simulink library "Batt_lib"  (Simulink 7.8)
settings: Solver=ode45  StartTime=0.0  StopTime=10.0  RelTol=1e-3
values from neighbouring files (symbols this model uses):
  batt_esr = (max_power*0.01)/(max_power/Vdc_nom)^2    [BES_init.m]
  C = IacRMS*18e-6    [BES_init.m]
  f = 60    [global_parameters.m]
  I_ki = 0.03    [BES_init.m]
  I_kp = 0.05    [BES_init.m]
  Iac_max = IGBT_currents(possible_currents(1))    [BES_init.m]
  Id_at_max = 3*max_pow*(2/3)/Vd_at_max    [BES_init.m]
  Iq_at_max = 3*max_pow*(2/3)/Vq_at_max    [BES_init.m]
  L = Vdc_nom/(IacRMS*0.2/(2/fs))    [BES_init.m]
  PLL_Ki = 0.001*30    (= 0.03)    [BES_init.m]
  PLL_Kp = .001*30    (= 0.03)    [BES_init.m]
  PLL_time_step = Ts    (= 8e-05)    [global_parameters.m]
  Roff = 1e7    (= 10000000)    [BES_init.m]
  Td_es_min = Ts    (= 8e-05)    [global_parameters.m]
  Tds = Ts    (= 8e-05)    [global_parameters.m]
  Ts = 80e-6    (= 8e-05)    [global_parameters.m]    (also in scopeBuffer.m)
  Vdc_max = IGBT_voltages(possible_voltages(1))    [BES_init.m]
undefined symbols (not defined in the file or in its folder): D, DiscIntNeverNeededParam
libraries: powerlib x17, simulink x14, simulink_extras x8, cstextras x3, rtio_generic_modbus x1, powerlib_extras x1
settings Model: Creator=re25624  LastModifiedBy=RE25624

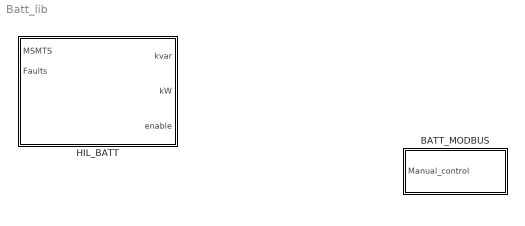
== system Batt_lib ==
  BATT_MODBUS : Subsystem
  HIL_BATT : Subsystem

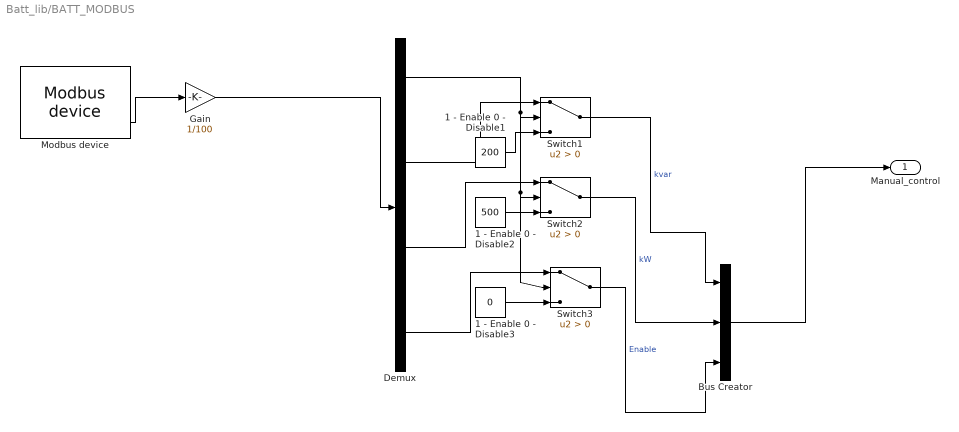
== system Batt_lib/BATT_MODBUS ==
  1 - Enable 0 - Disable1 : Constant  Value=200
  1 - Enable 0 - Disable2 : Constant  Value=500
  1 - Enable 0 - Disable3 : Constant  Value=0
  Bus Creator : BusCreator  Inputs=3
  Demux : Demux
  Gain : Gain  Gain=1/100
  Modbus device : rtio_generic_modbus/Modbus device  conf_name=batt_slave_cfg.opal  conf_name_mask=batt_slave_cfg.xls  sample_time=Ts
  Switch1 : Switch  Criteria=u2 > Threshold
  Switch2 : Switch  Criteria=u2 > Threshold
  Switch3 : Switch  Criteria=u2 > Threshold
  Manual_control : Outport
  wires:
  Bus Creator/1 -> Manual_control/1
  Switch3/1 -> Bus Creator/3  "Enable"
  Switch2/1 -> Bus Creator/2  "kW"
  Switch1/1 -> Bus Creator/1  "kvar"
  Demux/1 -> Switch3/2, Switch2/2, Switch1/2
  Demux/4 -> Switch3/1
  Demux/3 -> Switch2/1
  Demux/2 -> Switch1/1
  1 - Enable 0 - Disable3/1 -> Switch3/3
  1 - Enable 0 - Disable2/1 -> Switch2/3
  1 - Enable 0 - Disable1/1 -> Switch1/3
  Gain/1 -> Demux/1
  Modbus device/2 -> Gain/1

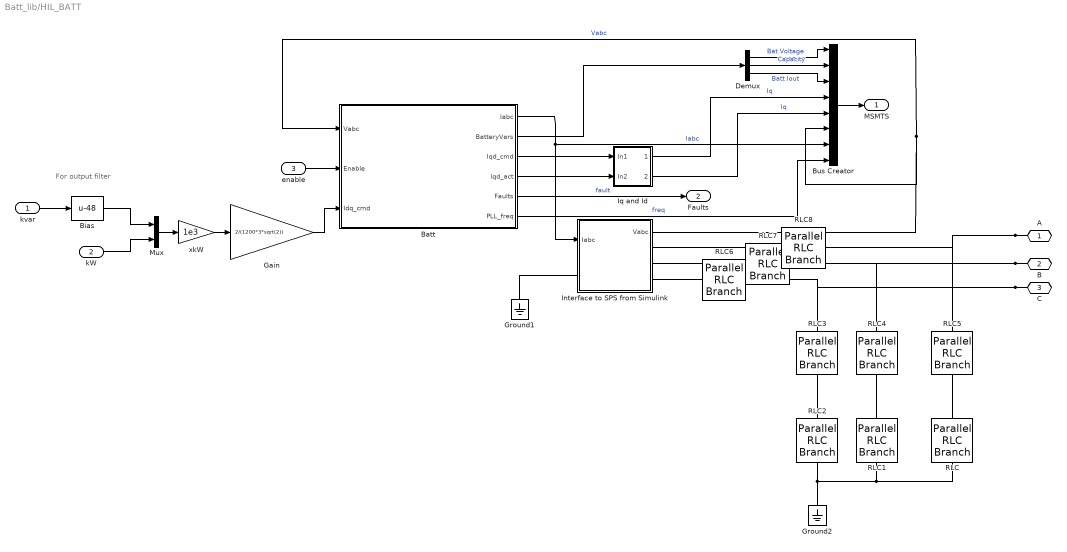
== system Batt_lib/HIL_BATT ==
  note: For output filter
  kvar : Inport
  kW : Inport  Port=2
  enable : Inport  Port=3
  Batt : Subsystem  mask(Battery Energy Storage System with AC inverter and Droop Control){max_power=4e6, batt_kWh=500, VacRMS=1200, Vdc_nom=4000}
      mask prompts: max_power "Peak Power (W)"; batt_kWh "Capacity (kWh)"; VacRMS "Grid Tie Line to Neutral Voltage (RMS)"; Vdc_nom "Nominal DC Battery Voltage"
      mask help: The block implements a battery energy storage system suitable for connecting to the grid. It responds to grid voltage changes by injecting current into the grid. The model is a non-switching average model.
      mask init:
      | global_parameters
      | BES_init
      mask Help:
      | This block will likely need a filter and transformer on it's output in order to connect to a high power line.
      | 
      | A unit delay block  on the Iabc output can help remove algebraic loops with minimal impact on simulation results.
      | 
      | 
      | Block Parameters:
      | Peak Power- Maximum power the unit can transfer.
      | Capacity- Amount of energy in the battery.
      | Grid Tie Line to Neutral Voltage- RMS voltage for the grid tie interface.
      | Nominal DC Battery Voltage- Open circuit full charge voltage.
      | Real Power Droop Gain- Ratio of Watts to Hz for injecting power to the grid in response to frequency changes.
      | Reactive Power Droop Gain- Ratio of kVars to RMS volts for injecting reactive power to the grid.
      | Droop Filter Cut Off- Fastest frequency that will be responded to for injecting power to the grid.
      | 
      | 
      | Block Connections:
      | Vabc- Grid voltage for each of the three phases.
      | Enable- Set to zero for no power.  Set to 1 to enable energy tranfer.
      | Iabc- Grid current for each of the three phases.  Connect to your grid.  Positive is into the grid.
      | Battery_vars- A vector of battery voltage, capacity, and current out of the battery.
      | Iqd_cmd- Commanded q and d axis currents.
      | Iqd_act- Actual q and d axis currents.
      mask Display:
      | image(imread('grid_storage_battery.jpg'))
      | color('white')
      | fprintf('%d kW Peak', max_power/1e3)
      | color('black')
      | port_label('input',1,'Vabc')
      | port_label('input',2,'Enable')
      | port_label('input',3,'Idq_cmd')
      | port_label('output',1,'Iabc')
      | port_label('output',2,'Battery_vars')
      | port_label('output',3,'Iqd_cmd')
      | port_label('output',4,'Iqd_act')
      | port_label('output',5,'Faults')
      | port_label('output',6,'Freq')
  Bias : Bias  Bias=-48
  Bus Creator : BusCreator  Inputs=8
  Demux : Demux  Outputs=3
  Gain : Gain  Gain=2/(1200*3*sqrt(2))
  Ground1 : powerlib/Elements/Ground  LConnTagsString=a
  Ground2 : powerlib/Elements/Ground  LConnTagsString=a
  Interface to SPS from Simulink : Subsystem
  Iq and Id : Subsystem
  Mux : Mux  Inputs=2
  "RLC " : powerlib/Elements/Parallel RLC Branch  LConnTagsString=a  RConnTagsString=__new0  BranchType=RLC  Resistance=500  Inductance=inf  SetiL0=off  InitialCurrent=0  Capacitance=10e-6  Setx0=off  InitialVoltage=0  Measurements=None
  RLC1 : powerlib/Elements/Parallel RLC Branch  LConnTagsString=a  RConnTagsString=__new0  BranchType=RLC  Resistance=500  Inductance=inf  SetiL0=off  InitialCurrent=0  Capacitance=10e-6  Setx0=off  InitialVoltage=0  Measurements=None
  RLC2 : powerlib/Elements/Parallel RLC Branch  LConnTagsString=a  RConnTagsString=__new0  BranchType=RLC  Resistance=500  Inductance=inf  SetiL0=off  InitialCurrent=0  Capacitance=10e-6  Setx0=off  InitialVoltage=0  Measurements=None
  RLC3 : powerlib/Elements/Parallel RLC Branch  LConnTagsString=a  RConnTagsString=__new0  BranchType=R  Resistance=10e-3  Inductance=inf  SetiL0=off  InitialCurrent=0  Capacitance=0  Setx0=off  InitialVoltage=0  Measurements=None
  RLC4 : powerlib/Elements/Parallel RLC Branch  LConnTagsString=a  RConnTagsString=__new0  BranchType=R  Resistance=10e-3  Inductance=inf  SetiL0=off  InitialCurrent=0  Capacitance=0  Setx0=off  InitialVoltage=0  Measurements=None
  RLC5 : powerlib/Elements/Parallel RLC Branch  LConnTagsString=a  RConnTagsString=__new0  BranchType=R  Resistance=10e-3  Inductance=inf  SetiL0=off  InitialCurrent=0  Capacitance=0  Setx0=off  InitialVoltage=0  Measurements=None
  RLC6 : powerlib/Elements/Parallel RLC Branch  LConnTagsString=a  RConnTagsString=__new0  BranchType=R  Resistance=20e-3  Inductance=inf  SetiL0=off  InitialCurrent=0  Capacitance=0  Setx0=off  InitialVoltage=0  Measurements=None
  RLC7 : powerlib/Elements/Parallel RLC Branch  LConnTagsString=a  RConnTagsString=__new0  BranchType=R  Resistance=20e-3  Inductance=inf  SetiL0=off  InitialCurrent=0  Capacitance=0  Setx0=off  InitialVoltage=0  Measurements=None
  RLC8 : powerlib/Elements/Parallel RLC Branch  LConnTagsString=a  RConnTagsString=__new0  BranchType=R  Resistance=20e-3  Inductance=inf  SetiL0=off  InitialCurrent=0  Capacitance=0  Setx0=off  InitialVoltage=0  Measurements=None
  xkW : Gain  Gain=1e3
  A : PMIOPort  Port=1  Side=Right
  B : PMIOPort  Port=2  Side=Right
  C : PMIOPort  Port=3  Side=Right
  MSMTS : Outport
  Faults : Outport  Port=2
  wires:
  Batt/5(Faults) -> Faults/1  "fault"
  Interface to SPS from Simulink/1(Vabc) -> Batt/1(Vabc), Bus Creator/6  "Vabc"
  Batt/2(BatteryVars) -> Demux/1
  Demux/2 -> Bus Creator/2  "Capacity"
  Demux/3 -> Bus Creator/3  "Batt Iout"
  Demux/1 -> Bus Creator/1  "Bat Voltage"
  Batt/3(Iqd_cmd) -> Iq and Id/1(In1)
  Batt/4(Iqd_act) -> Iq and Id/2(In2)
  Iq and Id/1(Out1) -> Bus Creator/4  "Iq"
  enable/1 -> Batt/2(Enable)
  Batt/1(Iabc) -> Bus Creator/7, Interface to SPS from Simulink/1(Iabc)  "Iabc"
  Gain/1 -> Batt/3(Idq_cmd)
  xkW/1 -> Gain/1
  Mux/1 -> xkW/1
  Iq and Id/2(Out2) -> Bus Creator/5  "Iq"
  Bus Creator/1 -> MSMTS/1
  kvar/1 -> Bias/1
  kW/1 -> Mux/2
  Batt/6(PLL_freq) -> Bus Creator/8  "freq"
  Bias/1 -> Mux/1
  connections:
  Interface to SPS from Simulink/LConn1 -- Ground1/LConn1
  Ground2/LConn1 -- RLC2/RConn1 -- "RLC "/RConn1 -- RLC1/RConn1
  A/RConn1 -- RLC8/LConn1 -- RLC5/LConn1
  B/RConn1 -- RLC7/LConn1 -- RLC4/LConn1
  C/RConn1 -- RLC6/LConn1 -- RLC3/LConn1
  RLC3/RConn1 -- RLC2/LConn1
  RLC4/RConn1 -- RLC1/LConn1
  RLC5/RConn1 -- "RLC "/LConn1
  RLC6/RConn1 -- Interface to SPS from Simulink/RConn3
  Interface to SPS from Simulink/RConn2 -- RLC7/RConn1
  Interface to SPS from Simulink/RConn1 -- RLC8/RConn1

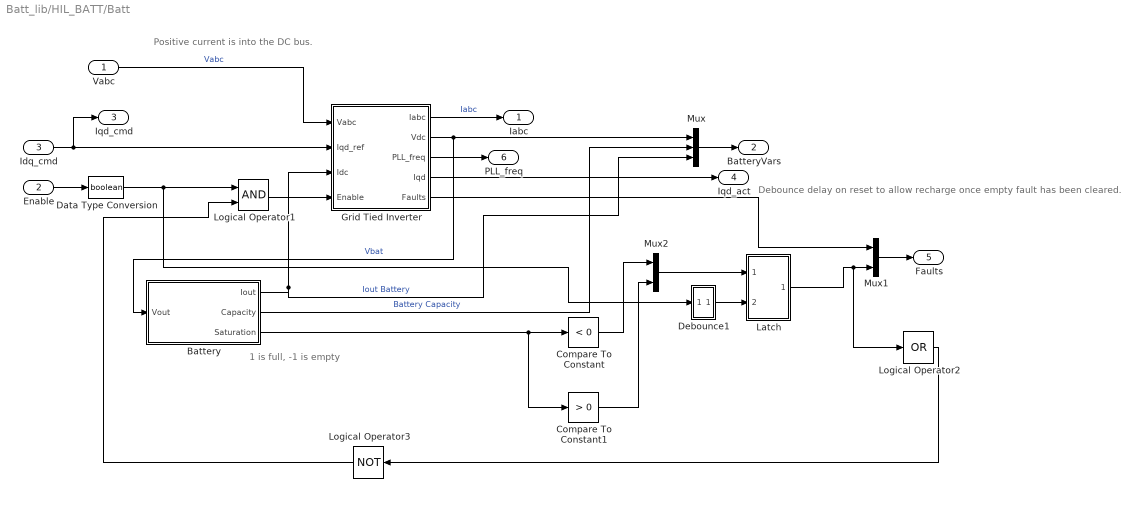
== system Batt_lib/HIL_BATT/Batt ==
  note: Debounce delay on reset to allow recharge once empty fault has been cleared.
  note: 1 is full, -1 is empty
  note: Positive current is into the DC bus.
  Vabc : Inport
  Enable : Inport  Port=2  OutDataTypeStr=double
  Idq_cmd : Inport  Port=3
  Battery : Subsystem  mask(Very simple battery model.  ){kWh=batt_kWh, esr=batt_esr, Vdc_nom=Vdc_nom}
      mask prompts: kWh "Capacity  (kWh)"; esr "Output Resistance (Ohms)"; Vdc_nom "Open Circuit Voltage"
      mask help: Model integrates charge and stops at the rated capacity. When charge is all removed the current drops to zero.
      mask Help: This model views the battery as a voltage source with a fixed equivalent series resistance and a perfect integrator for capacity.
  Compare To Constant : simulink/Logic and Bit Operations/Compare To Constant  relop=<  const=0  OutDataTypeStr=boolean
  Compare To Constant1 : simulink/Logic and Bit Operations/Compare To Constant  relop=>  const=0  OutDataTypeStr=boolean
  Data Type Conversion : DataTypeConversion  OutDataTypeStr=boolean
  Debounce1 : Subsystem  mask{Ts=Ts, Td=0.1}
      mask prompts: Ts "Sample Time"; Td "Debounce Time"
  Grid Tied Inverter : Subsystem
  Latch : Subsystem
  Logical Operator1 : Logic  AllPortsSameDT=off  OutDataTypeStr=boolean
  Logical Operator2 : Logic  Operator=OR  Inputs=1  AllPortsSameDT=off  OutDataTypeStr=boolean
  Logical Operator3 : Logic  Operator=NOT  AllPortsSameDT=off  OutDataTypeStr=boolean
  Mux : Mux  Inputs=3
  Mux1 : Mux  Inputs=2
  Mux2 : Mux  Inputs=2
  Iabc : Outport
  BatteryVars : Outport  Port=2
  Iqd_cmd : Outport  Port=3
  Iqd_act : Outport  Port=4
  Faults : Outport  Port=5
  PLL_freq : Outport  Port=6
  wires:
  Debounce1/1(Out1) -> Latch/2(Reset)
  Mux2/1 -> Latch/1(In1)
  Latch/1(Out1) -> Logical Operator2/1, Mux1/2
  Grid Tied Inverter/5(Faults) -> Mux1/1
  Logical Operator3/1 -> Logical Operator1/2
  Logical Operator2/1 -> Logical Operator3/1
  Data Type Conversion/1 -> Debounce1/1(In1), Logical Operator1/1
  Logical Operator1/1 -> Grid Tied Inverter/4(Enable)
  Compare To Constant1/1 -> Mux2/2
  Compare To Constant/1 -> Mux2/1
  Battery/3(Saturation) -> Compare To Constant1/1, Compare To Constant/1
  Mux1/1 -> Faults/1
  Enable/1 -> Data Type Conversion/1
  Idq_cmd/1 -> Iqd_cmd/1, Grid Tied Inverter/2(Iqd_ref)
  Grid Tied Inverter/4(Iqd) -> Iqd_act/1
  Mux/1 -> BatteryVars/1
  Grid Tied Inverter/1(Iabc) -> Iabc/1  "Iabc"
  Battery/2(Capacity) -> Mux/2  "Battery Capacity"
  Battery/1(Iout) -> Mux/3, Grid Tied Inverter/3(Idc)  "Iout Battery"
  Grid Tied Inverter/2(Vdc) -> Battery/1(Vout), Mux/1  "Vbat"
  Vabc/1 -> Grid Tied Inverter/1(Vabc)  "Vabc"
  Grid Tied Inverter/3(PLL_freq) -> PLL_freq/1

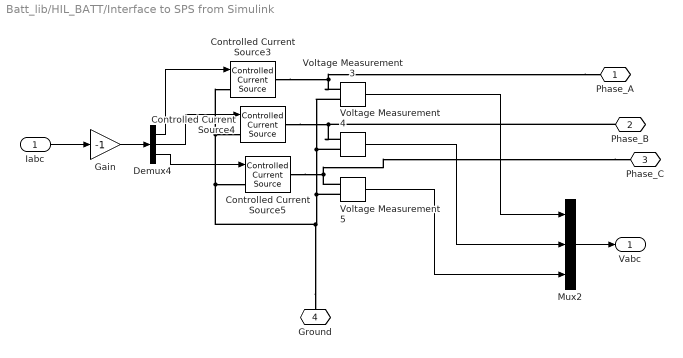
== system Batt_lib/HIL_BATT/Interface to SPS from Simulink ==
  Iabc : Inport
  Controlled Current Source3 : powerlib/Electrical Sources/Controlled Current Source  Initialize=on  Source_Type=AC  Amplitude=0  Phase=0  Frequency=0  Measurements=None
  Controlled Current Source4 : powerlib/Electrical Sources/Controlled Current Source  Initialize=on  Source_Type=AC  Amplitude=0  Phase=0  Frequency=0  Measurements=None
  Controlled Current Source5 : powerlib/Electrical Sources/Controlled Current Source  Initialize=on  Source_Type=AC  Amplitude=0  Phase=0  Frequency=0  Measurements=None
  Demux4 : Demux  Outputs=3
  Gain : Gain  Gain=-1
  Mux2 : Mux  Inputs=3
  Voltage Measurement3 : powerlib/Measurements/Voltage Measurement  PhasorSimulation=off  OutputType=Complex  PSBequivalent=0
  Voltage Measurement4 : powerlib/Measurements/Voltage Measurement  PhasorSimulation=off  OutputType=Complex  PSBequivalent=0
  Voltage Measurement5 : powerlib/Measurements/Voltage Measurement  PhasorSimulation=off  OutputType=Complex  PSBequivalent=0
  Phase_A : PMIOPort  Port=1  Side=Right
  Phase_B : PMIOPort  Port=2  Side=Right
  Phase_C : PMIOPort  Port=3  Side=Right
  Ground : PMIOPort  Port=4  Side=Left
  Vabc : Outport
  wires:
  Gain/1 -> Demux4/1
  Voltage Measurement3/1 -> Mux2/1
  Mux2/1 -> Vabc/1
  Iabc/1 -> Gain/1
  Demux4/3 -> Controlled Current Source5/1
  Demux4/2 -> Controlled Current Source4/1
  Demux4/1 -> Controlled Current Source3/1
  Voltage Measurement4/1 -> Mux2/2
  Voltage Measurement5/1 -> Mux2/3
  connections:
  Phase_B/RConn1 -- Controlled Current Source4/RConn1 -- Voltage Measurement4/LConn1
  Ground/RConn1 -- Voltage Measurement5/LConn2 -- Voltage Measurement3/LConn2 -- Voltage Measurement4/LConn2 -- Controlled Current Source4/LConn1 -- Controlled Current Source3/LConn1 -- Controlled Current Source5/LConn1
  Phase_A/RConn1 -- Controlled Current Source3/RConn1 -- Voltage Measurement3/LConn1
  Phase_C/RConn1 -- Controlled Current Source5/RConn1 -- Voltage Measurement5/LConn1

== system Batt_lib/HIL_BATT/Iq and Id ==
  In1 : Inport
  In2 : Inport  Port=2
  Demux1 : Demux  Outputs=2
  Demux2 : Demux  Outputs=2
  Mux : Mux  Inputs=2
  Mux1 : Mux  Inputs=2
  Out1 : Outport
  Out2 : Outport  Port=2
  wires:
  Demux1/2 -> Mux1/1  "Id_cmd"
  Demux2/1 -> Mux/2  "Iq_act"
  Demux1/1 -> Mux/1  "Iq_cmd"
  Demux2/2 -> Mux1/2  "Id_act"
  In1/1 -> Demux1/1
  In2/1 -> Demux2/1
  Mux/1 -> Out1/1
  Mux1/1 -> Out2/1

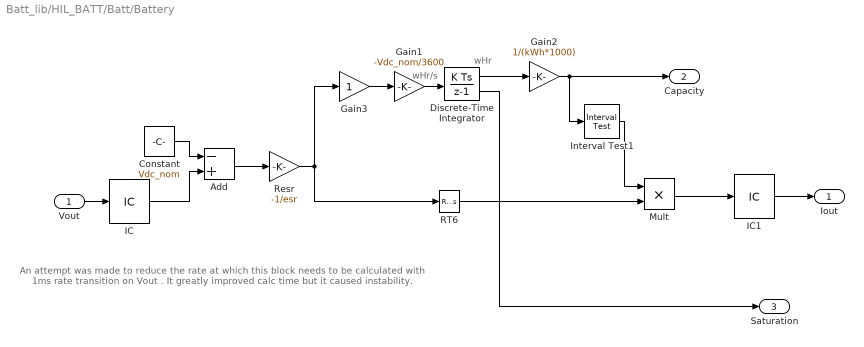
== system Batt_lib/HIL_BATT/Batt/Battery ==
  note: wHr
  note: wHr/s
  note: An attempt was made to reduce the rate at which this block
      | needs to be calculated with 1ms rate transition on
      | Vout .  It greatly improved calc time but it caused instability.
  Vout : Inport
  Add : Sum  Inputs=-+
  Constant : Constant  Value=Vdc_nom  SampleTime=Tds
  Discrete-Time Integrator : DiscreteIntegrator  InitialCondition=kWh*0.5*1000  InitialConditionMode=State only (most efficient)  SampleTime=Tds  LimitOutput=on  UpperSaturationLimit=(kWh*1000)  LowerSaturationLimit=0  ShowSaturationPort=on  ICPrevOutput=DiscIntNeverNeededParam  ICPrevScaledInput=DiscIntNeverNeededParam
  Gain1 : Gain  Gain=-Vdc_nom/3600
  Gain2 : Gain  Gain=1/(kWh*1000)
  Gain3 : Gain
  IC : InitialCondition  Value=Vdc_nom
  IC1 : InitialCondition  Value=0
  Interval Test1 : simulink/Logic and Bit Operations/Interval Test  IntervalClosedRight=on  uplimit=1  IntervalClosedLeft=on  lowlimit=0  OutDataTypeStr=boolean
  Mult : Product  Inputs=**
  RT6 : RateTransition  OutPortSampleTime=Tds
  Resr : Gain  Gain=-1/esr
  Iout : Outport
  Capacity : Outport  Port=2
  Saturation : Outport  Port=3
  wires:
  Discrete-Time Integrator/2 -> Saturation/1
  Gain3/1 -> Gain1/1
  RT6/1 -> Mult/2
  IC1/1 -> Iout/1
  IC/1 -> Add/2
  Discrete-Time Integrator/1 -> Gain2/1
  Gain2/1 -> Interval Test1/1, Capacity/1
  Resr/1 -> Gain3/1, RT6/1
  Mult/1 -> IC1/1
  Vout/1 -> IC/1
  Interval Test1/1 -> Mult/1
  Gain1/1 -> Discrete-Time Integrator/1
  Add/1 -> Resr/1
  Constant/1 -> Add/1

== system Batt_lib/HIL_BATT/Batt/Debounce1 ==
  In1 : Inport
  Compare To Constant1 : simulink/Logic and Bit Operations/Compare To Constant  relop=>  const=1  OutDataTypeStr=boolean
  Discrete-Time Integrator : DiscreteIntegrator  IntegratorMethod=Accumulation: Forward Euler  gainval=Ts/Td  ExternalReset=level  SampleTime=Ts  OutDataTypeStr=double  UpperSaturationLimit=1.001  LowerSaturationLimit=0  ICPrevOutput=DiscIntNeverNeededParam  ICPrevScaledInput=DiscIntNeverNeededParam
  Logical Operator : Logic  Operator=NOT  AllPortsSameDT=off  OutDataTypeStr=boolean
  Out1 : Outport
  wires:
  Discrete-Time Integrator/1 -> Compare To Constant1/1
  Logical Operator/1 -> Discrete-Time Integrator/2
  In1/1 -> Logical Operator/1, Discrete-Time Integrator/1
  Compare To Constant1/1 -> Out1/1

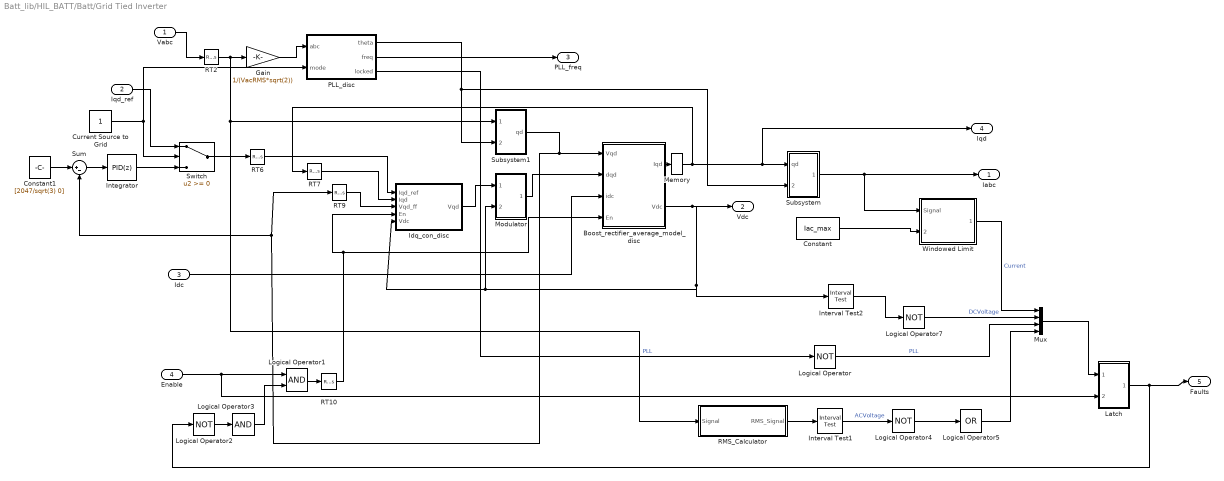
== system Batt_lib/HIL_BATT/Batt/Grid Tied Inverter ==
  Vabc : Inport
  Iqd_ref : Inport  Port=2
  Idc : Inport  Port=3
  Enable : Inport  Port=4
  Boost_rectifier_average_model_disc : Subsystem  mask{C=C, L=L, Roff=Roff, Vdc_nom=Vdc_nom}
      mask prompts: C "DC Bus Capacitance"; L "Boost Inductor"; Roff "Switch resistance when off"; Vdc_nom "Nominal DC Bus Voltage"
      mask init:
      | global_parameters
  Constant : Constant  Value=Iac_max
  Constant1 : Constant  Value=[2047/sqrt(3) 0]
  Current Source to Grid : Constant
  Gain : Gain  Gain=1/(VacRMS*sqrt(2))
  Idq_con_disc : Subsystem  mask{L=L, iq_max=Iq_at_max, id_max=Id_at_max, kp=I_kp, ki=I_ki, Vdc_nom=Vdc_nom}
      mask prompts: L "Boost Inductor"; iq_max "Maximum Iq"; id_max "Maximum Id"; kp "Proportional Gain"; ki "Integral Gain"; Vdc_nom "Nominal DC Bus Voltage"
      mask init:
      | global_parameters
  Integrator : simulink/Continuous/PID Controller  Controller=PID  TimeDomain=Discrete-time  SampleTime=Ts  IntegratorMethod=Forward Euler  FilterMethod=Forward Euler  Form=Parallel  P=2  I=0  D=0  N=100  InitialConditionSource=internal  InitialConditionForIntegrator=0  InitialConditionForFilter=0  ExternalReset=none  LimitOutput=on  UpperSaturationLimit=2000  LowerSaturationLimit=-2000  LinearizeAsGain=off  AntiWindupMode=clamping  Kb=1  TrackingMode=off  Kt=1  PParamMin=[]  PParamMax=[]  IParamMin=[]  IParamMax=[]  DParamMin=[]  DParamMax=[]  NParamMin=[]  NParamMax=[]  KbParamMin=[]  KbParamMax=[]  KtParamMin=[]  KtParamMax=[]  POutMin=[]  POutMax=[]  IOutMin=[]  IOutMax=[]  DOutMin=[]  DOutMax=[]  NOutMin=[]  NOutMax=[]  KbOutMin=[]  KbOutMax=[]  KtOutMin=[]  KtOutMax=[]  IntegratorOutMin=[]  IntegratorOutMax=[]  FilterOutMin=[]  FilterOutMax=[]  SumOutMin=[]  SumOutMax=[]  SumI1OutMin=[]  SumI1OutMax=[]  SumI2OutMin=[]  SumI2OutMax=[]  SumI3OutMin=[]  SumI3OutMax=[]  SumDOutMin=[]  SumDOutMax=[]  SaturationOutMin=[]  SaturationOutMax=[]  IntegratorContinuousStateAttributes=''  IntegratorStateMustResolveToSignalObject=off  IntegratorRTWStateStorageClass=Auto  FilterContinuousStateAttributes=''  FilterStateMustResolveToSignalObject=off  FilterRTWStateStorageClass=Auto
  Interval Test1 : simulink/Logic and Bit Operations/Interval Test  IntervalClosedRight=on  uplimit=VacRMS*1.15  IntervalClosedLeft=on  lowlimit=VacRMS*0.85  OutDataTypeStr=boolean
  Interval Test2 : simulink/Logic and Bit Operations/Interval Test  IntervalClosedRight=on  uplimit=Vdc_max  IntervalClosedLeft=on  lowlimit=2000  OutDataTypeStr=boolean
  Latch : Subsystem
  Logical Operator{,2,4,7} (4 alike) : Logic  Operator=NOT  AllPortsSameDT=off  OutDataTypeStr=boolean
  Logical Operator1 : Logic  AllPortsSameDT=off  OutDataTypeStr=boolean
  Logical Operator3 : Logic  Inputs=1  AllPortsSameDT=off  OutDataTypeStr=boolean
  Logical Operator5 : Logic  Operator=OR  Inputs=1  AllPortsSameDT=off  OutDataTypeStr=boolean
  Memory : Memory  InheritSampleTime=on
  Modulator : Subsystem
  Mux : Mux
  PLL_disc : Subsystem  mask{PLL_Kp=PLL_Kp, PLL_Ki=PLL_Ki, PLL_freq_range=0.25, PLL_lock_window=0.1}
      mask prompts: PLL_Kp "Proportional Gain"; PLL_Ki "Integral Gain"; PLL_freq_range "PLL Frequency Range"; PLL_lock_window "PLL Lock Window"
  RMS_Calculator : Subsystem
  RT{2,6..7,9..10} (5 alike) : RateTransition  OutPortSampleTime=Td_es_min
  Subsystem : Subsystem
  Subsystem1 : Subsystem
  Sum : Sum  Inputs=|+-
  Switch : Switch
  Windowed Limit : Subsystem
  Iabc : Outport
  Vdc : Outport  Port=2
  PLL_freq : Outport  Port=3
  Iqd : Outport  Port=4
  Faults : Outport  Port=5
  wires:
  Constant1/1 -> Sum/1
  Sum/1 -> Integrator/1
  Current Source to Grid/1 -> PLL_disc/2(mode), Switch/2
  Iqd_ref/1 -> Switch/1
  Integrator/1 -> Switch/3
  Switch/1 -> RT6/1
  Logical Operator7/1 -> Mux/2  "DCVoltage"
  Memory/1 -> RT7/1, Iqd/1, Subsystem/1(qd)
  RT10/1 -> Idq_con_disc/4(En), Boost_rectifier_average_model_disc/4(En)
  RT9/1 -> Idq_con_disc/3(Vqd_ff)
  RT6/1 -> Idq_con_disc/1(Iqd_ref)
  RT2/1 -> Gain/1, Subsystem1/1(abc), RMS_Calculator/1(Signal)
  Vabc/1 -> RT2/1
  PLL_disc/1(theta) -> Subsystem/2(theta), Subsystem1/2(theta)
  Enable/1 -> Latch/2(Reset), Logical Operator1/1
  Gain/1 -> PLL_disc/1(abc)
  Logical Operator/1 -> Mux/3  "PLL"
  PLL_disc/3(locked) -> Logical Operator/1  "PLL"
  Modulator/1(dqd) -> Boost_rectifier_average_model_disc/2(dqd)
  PLL_disc/2(freq) -> PLL_freq/1
  Interval Test2/1 -> Logical Operator7/1
  Windowed Limit/1(TestOut) -> Mux/1  "Current"
  Constant/1 -> Windowed Limit/2(Threshold)
  Logical Operator1/1 -> RT10/1
  Idq_con_disc/1(Vqd) -> Modulator/1(Vqd)
  Subsystem/1(abc) -> Iabc/1, Windowed Limit/1(Signal)
  Boost_rectifier_average_model_disc/1(Iqd) -> Memory/1
  Subsystem1/1(qd) -> Sum/2, RT9/1, Boost_rectifier_average_model_disc/1(Vqd)
  Logical Operator2/1 -> Logical Operator3/1
  Logical Operator3/1 -> Logical Operator1/2
  RMS_Calculator/1(RMS_Signal) -> Interval Test1/1
  Interval Test1/1 -> Logical Operator4/1  "ACVoltage"
  Logical Operator4/1 -> Logical Operator5/1
  Logical Operator5/1 -> Mux/4
  Boost_rectifier_average_model_disc/2(Vdc) -> Vdc/1, Interval Test2/1, Idq_con_disc/5(Vdc), Modulator/2(Vdc)
  Idc/1 -> Boost_rectifier_average_model_disc/3(idc)
  RT7/1 -> Idq_con_disc/2(Iqd)
  Mux/1 -> Latch/1(In1)
  Latch/1(Out1) -> Logical Operator2/1, Faults/1

== system Batt_lib/HIL_BATT/Batt/Latch ==
  In1 : Inport
  Reset : Inport  Port=2
  Demux : Demux  Outputs=2
  Logical Operator6 : Logic  Operator=NOT  AllPortsSameDT=off  OutDataTypeStr=boolean
  Mux : Mux  Inputs=2
  S-R Flip-Flop : simulink_extras/Flip Flops/S-R Flip-Flop  initial_condition=0
  S-R Flip-Flop1 : simulink_extras/Flip Flops/S-R Flip-Flop  initial_condition=0
  Out1 : Outport
  wires:
  Logical Operator6/1 -> S-R Flip-Flop1/2, S-R Flip-Flop/2
  Reset/1 -> Logical Operator6/1
  Demux/2 -> S-R Flip-Flop1/1
  S-R Flip-Flop1/1 -> Mux/2  "Ib"
  In1/1 -> Demux/1
  Demux/1 -> S-R Flip-Flop/1
  Mux/1 -> Out1/1  "Faults"
  S-R Flip-Flop/1 -> Mux/1  "Ia"

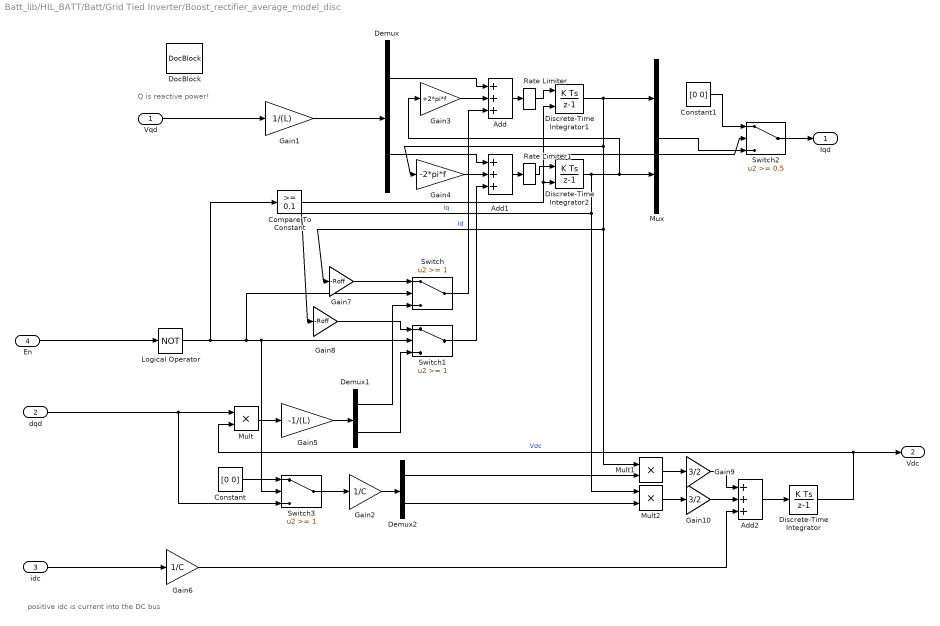
== system Batt_lib/HIL_BATT/Batt/Grid Tied Inverter/Boost_rectifier_average_model_disc ==
  note: Q is reactive power!
  note: positive idc is current into the DC bus
  Vqd : Inport
  dqd : Inport  Port=2  PortDimensions=2
  idc : Inport  Port=3
  En : Inport  Port=4  OutDataTypeStr=boolean
  Add : Sum  Inputs=+++
  Add1 : Sum  Inputs=+++
  Add2 : Sum  Inputs=+++
  Compare To Constant : simulink/Logic and Bit Operations/Compare To Constant  relop=>=  const=0.1  OutDataTypeStr=uint8
  Constant : Constant  Value=[0 0]
  Constant1 : Constant  Value=[0 0]
  Demux : Demux  Outputs=2
  Demux1 : Demux  Outputs=2
  Demux2 : Demux  Outputs=2
  Discrete-Time Integrator : DiscreteIntegrator  InitialCondition=Vdc_nom  InitialConditionMode=State only (most efficient)  SampleTime=Tds  ICPrevOutput=DiscIntNeverNeededParam  ICPrevScaledInput=DiscIntNeverNeededParam
  Discrete-Time Integrator1 : DiscreteIntegrator  ExternalReset=rising  InitialConditionMode=State only (most efficient)  SampleTime=Tds  ICPrevOutput=DiscIntNeverNeededParam  ICPrevScaledInput=DiscIntNeverNeededParam
  Discrete-Time Integrator2 : DiscreteIntegrator  ExternalReset=rising  InitialConditionMode=State only (most efficient)  SampleTime=Tds  ICPrevOutput=DiscIntNeverNeededParam  ICPrevScaledInput=DiscIntNeverNeededParam
  DocBlock : simulink/Model-Wide Utilities/DocBlock  DocumentType=Text
  Gain1 : Gain  Gain=1/(L)
  Gain10 : Gain  Gain=3/2
  Gain2 : Gain  Gain=1/C
  Gain3 : Gain  Gain=+2*pi*f
  Gain4 : Gain  Gain=-2*pi*f
  Gain5 : Gain  Gain=-1/(L)
  Gain6 : Gain  Gain=1/C
  Gain7 : Gain  Gain=-Roff
  Gain8 : Gain  Gain=-Roff
  Gain9 : Gain  Gain=3/2
  Logical Operator : Logic  Operator=NOT  AllPortsSameDT=off  OutDataTypeStr=boolean
  Mult : Product  Inputs=**
  Mult1 : Product  Inputs=**
  Mult2 : Product  Inputs=**
  Mux : Mux  Inputs=2
  Rate Limiter : RateLimiter  RisingSlewLimit=1e6  FallingSlewLimit=-1e6  SampleTimeMode=inherited
  Rate Limiter1 : RateLimiter  RisingSlewLimit=1e6  FallingSlewLimit=-1e6  SampleTimeMode=inherited
  Switch : Switch  Threshold=1
  Switch1 : Switch  Threshold=1
  Switch2 : Switch  Threshold=0.5
  Switch3 : Switch  Threshold=1
  Iqd : Outport
  Vdc : Outport  Port=2
  wires:
  Rate Limiter1/1 -> Discrete-Time Integrator2/1
  Rate Limiter/1 -> Discrete-Time Integrator1/1
  Add1/1 -> Rate Limiter1/1
  Gain8/1 -> Switch1/1
  Discrete-Time Integrator2/1 -> Mux/2, Gain3/1, Mult2/1, Gain8/1  "Iq"
  Demux1/2 -> Switch1/3
  Mult1/1 -> Gain9/1
  Switch1/1 -> Add1/3
  Add/1 -> Rate Limiter/1
  Switch/1 -> Add/3
  Gain1/1 -> Demux/1
  Gain5/1 -> Demux1/1
  Mult2/1 -> Gain10/1
  Constant/1 -> Switch3/1
  Gain9/1 -> Add2/1
  Demux2/2 -> Mult2/2
  idc/1 -> Gain6/1
  Mult/1 -> Gain5/1
  Add2/1 -> Discrete-Time Integrator/1
  Gain7/1 -> Switch/1
  Demux/1 -> Add/1
  En/1 -> Logical Operator/1
  Discrete-Time Integrator1/1 -> Mux/1, Gain4/1, Mult1/1, Gain7/1  "Id"
  Switch3/1 -> Gain2/1
  Logical Operator/1 -> Compare To Constant/1, Switch/2, Switch1/2, Switch3/2
  Gain10/1 -> Add2/2
  Gain6/1 -> Add2/3
  Gain2/1 -> Demux2/1
  Demux1/1 -> Switch/3
  Gain4/1 -> Add1/2
  Gain3/1 -> Add/2
  Demux2/1 -> Mult1/2
  Demux/2 -> Add1/1
  Discrete-Time Integrator/1 -> Vdc/1, Mult/2  "Vdc"
  dqd/1 -> Mult/1, Switch3/3
  Vqd/1 -> Gain1/1
  Compare To Constant/1 -> Discrete-Time Integrator1/2, Switch2/2, Discrete-Time Integrator2/2
  Switch2/1 -> Iqd/1
  Constant1/1 -> Switch2/1
  Mux/1 -> Switch2/3

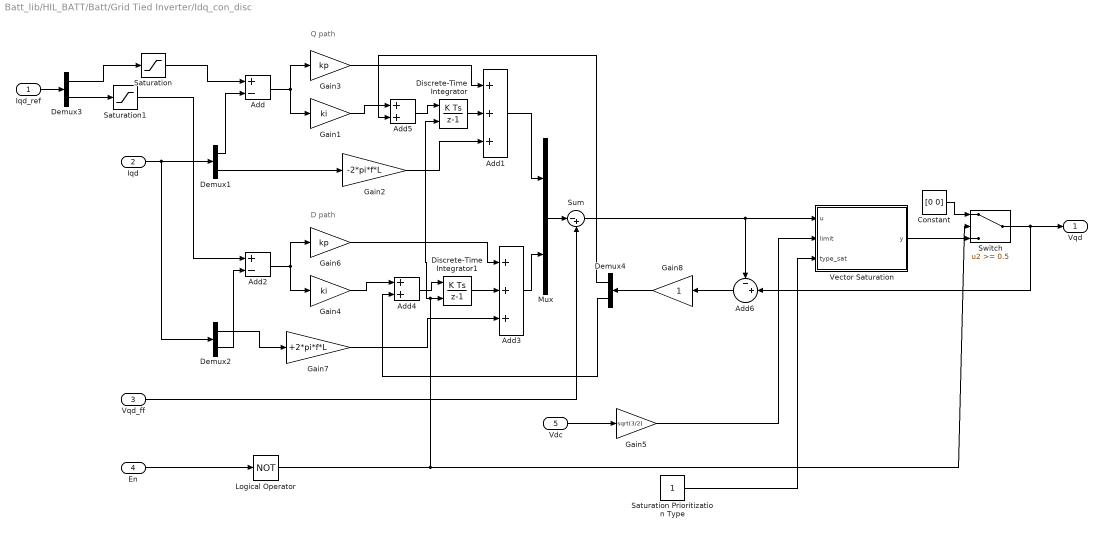
== system Batt_lib/HIL_BATT/Batt/Grid Tied Inverter/Idq_con_disc ==
  note: Q path
  note: D path
  Iqd_ref : Inport
  Iqd : Inport  Port=2
  Vqd_ff : Inport  Port=3  PortDimensions=2
  En : Inport  Port=4  OutDataTypeStr=boolean  PortDimensions=1
  Vdc : Inport  Port=5  PortDimensions=1
  Add : Sum  Inputs=+-
  Add1 : Sum  Inputs=+++
  Add2 : Sum  Inputs=+-
  Add3 : Sum  Inputs=+++
  Add4 : Sum
  Add5 : Sum
  Add6 : Sum  Inputs=-+|
  Constant : Constant  Value=[0 0]
  Demux{1..4} (4 alike) : Demux  Outputs=2
  Discrete-Time Integrator : DiscreteIntegrator  ExternalReset=level  InitialConditionMode=State only (most efficient)  SampleTime=Td_es_min  ICPrevOutput=DiscIntNeverNeededParam  ICPrevScaledInput=DiscIntNeverNeededParam
  Discrete-Time Integrator1 : DiscreteIntegrator  ExternalReset=level  InitialConditionMode=State only (most efficient)  SampleTime=Td_es_min  ICPrevOutput=DiscIntNeverNeededParam  ICPrevScaledInput=DiscIntNeverNeededParam
  Gain1 : Gain  Gain=ki
  Gain2 : Gain  Gain=-2*pi*f*L
  Gain3 : Gain  Gain=kp
  Gain4 : Gain  Gain=ki
  Gain5 : Gain  Gain=sqrt(3/2)
  Gain6 : Gain  Gain=kp
  Gain7 : Gain  Gain=+2*pi*f*L
  Gain8 : Gain
  Logical Operator : Logic  Operator=NOT  AllPortsSameDT=off  OutDataTypeStr=boolean
  Mux : Mux  Inputs=2
  Saturation : Saturate  UpperLimit=iq_max  LowerLimit=-iq_max
  Saturation Prioritization Type : Constant
  Saturation1 : Saturate  UpperLimit=id_max  LowerLimit=-id_max
  Sum : Sum  Inputs=|-+
  Switch : Switch  Threshold=0.5
  Vector Saturation : MATLAB Function  TreatAsAtomicUnit=on
  Vqd : Outport
  wires:
  Add/1 -> Gain1/1, Gain3/1
  Gain6/1 -> Add3/1
  Demux4/2 -> Add4/2
  Mux/1 -> Sum/1
  Discrete-Time Integrator1/1 -> Add3/2
  Gain7/1 -> Add3/3
  Demux2/2 -> Add2/2
  Add3/1 -> Mux/2
  En/1 -> Logical Operator/1
  Gain1/1 -> Add5/1
  Gain2/1 -> Add1/3
  Demux3/2 -> Saturation1/1
  Discrete-Time Integrator/1 -> Add1/2
  Iqd/1 -> Demux2/1, Demux1/1
  Add4/1 -> Discrete-Time Integrator1/1
  Demux3/1 -> Saturation/1
  Add5/1 -> Discrete-Time Integrator/1
  Gain4/1 -> Add4/1
  Add1/1 -> Mux/1
  Sum/1 -> Vector Saturation/1(u), Add6/1
  Gain3/1 -> Add1/1
  Demux1/1 -> Add/2
  Demux1/2 -> Gain2/1
  Add2/1 -> Gain4/1, Gain6/1
  Gain8/1 -> Demux4/1
  Iqd_ref/1 -> Demux3/1
  Saturation1/1 -> Add2/1
  Saturation/1 -> Add/1
  Demux4/1 -> Add5/2
  Demux2/1 -> Gain7/1
  Vqd_ff/1 -> Sum/2
  Saturation Prioritization Type/1 -> Vector Saturation/3(type_sat)
  Gain5/1 -> Vector Saturation/2(limit)
  Add6/1 -> Gain8/1
  Vdc/1 -> Gain5/1
  Switch/1 -> Vqd/1, Add6/2
  Logical Operator/1 -> Discrete-Time Integrator/2, Discrete-Time Integrator1/2, Switch/2
  Vector Saturation/1(y) -> Switch/3
  Constant/1 -> Switch/1

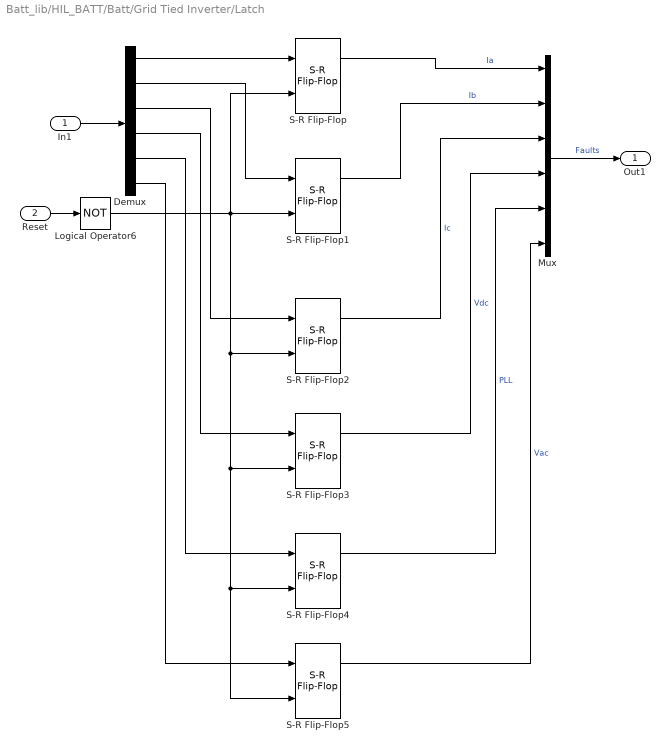
== system Batt_lib/HIL_BATT/Batt/Grid Tied Inverter/Latch ==
  In1 : Inport
  Reset : Inport  Port=2
  Demux : Demux  Outputs=6
  Logical Operator6 : Logic  Operator=NOT  AllPortsSameDT=off  OutDataTypeStr=boolean
  Mux : Mux  Inputs=6
  S-R Flip-Flop{,1..5} (6 alike) : simulink_extras/Flip Flops/S-R Flip-Flop  initial_condition=0
  Out1 : Outport
  wires:
  Logical Operator6/1 -> S-R Flip-Flop1/2, S-R Flip-Flop/2, S-R Flip-Flop2/2, S-R Flip-Flop3/2, S-R Flip-Flop4/2, S-R Flip-Flop5/2
  Reset/1 -> Logical Operator6/1
  Demux/2 -> S-R Flip-Flop1/1
  S-R Flip-Flop1/1 -> Mux/2  "Ib"
  In1/1 -> Demux/1
  Demux/1 -> S-R Flip-Flop/1
  Mux/1 -> Out1/1  "Faults"
  S-R Flip-Flop/1 -> Mux/1  "Ia"
  S-R Flip-Flop2/1 -> Mux/3  "Ic"
  Demux/3 -> S-R Flip-Flop2/1
  Demux/4 -> S-R Flip-Flop3/1
  Demux/5 -> S-R Flip-Flop4/1
  Demux/6 -> S-R Flip-Flop5/1
  S-R Flip-Flop3/1 -> Mux/4  "Vdc"
  S-R Flip-Flop4/1 -> Mux/5  "PLL"
  S-R Flip-Flop5/1 -> Mux/6  "Vac"

== system Batt_lib/HIL_BATT/Batt/Grid Tied Inverter/Modulator ==
  Vqd : Inport
  Vdc : Inport  Port=2
  Delay : Delay  DelayLength=1  InitialCondition=[0 0]  SampleTime=Td_es_min
  IC : InitialCondition  Value=Vdc_nom
  Mult1 : Product  Inputs=*/
  Saturation : Saturate  UpperLimit=1  LowerLimit=-1
  dqd : Outport
  wires:
  Delay/1 -> dqd/1
  IC/1 -> Mult1/2
  Vdc/1 -> IC/1
  Vqd/1 -> Mult1/1
  Saturation/1 -> Delay/1
  Mult1/1 -> Saturation/1

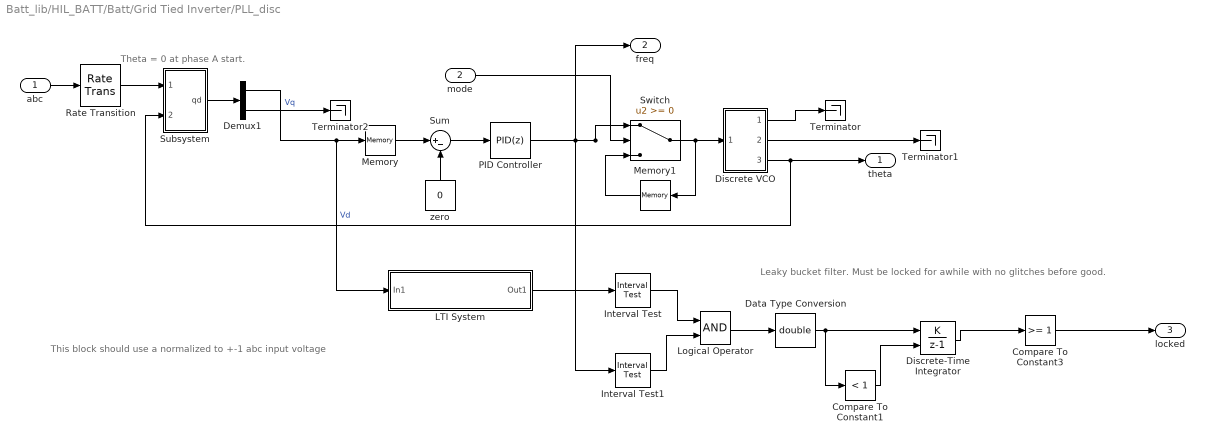
== system Batt_lib/HIL_BATT/Batt/Grid Tied Inverter/PLL_disc ==
  note: This block should use a normalized to +-1 abc input voltage
  note: Theta = 0 at phase A start.
  note: Leaky bucket filter. Must be locked for awhile with no glitches before good.
  abc : Inport  PortDimensions=3
  mode : Inport  Port=2
  Compare To Constant1 : simulink/Logic and Bit Operations/Compare To Constant  relop=<  const=1  OutDataTypeStr=boolean
  Compare To Constant3 : simulink/Logic and Bit Operations/Compare To Constant  relop=>=  const=1  OutDataTypeStr=boolean
  Data Type Conversion : DataTypeConversion  OutDataTypeStr=double
  Demux1 : Demux  Outputs=2
  Discrete VCO : Subsystem
  Discrete-Time Integrator : DiscreteIntegrator  IntegratorMethod=Accumulation: Forward Euler  gainval=Td_es_min/0.5  ExternalReset=rising  SampleTime=Td_es_min  LimitOutput=on  UpperSaturationLimit=1  LowerSaturationLimit=0  ICPrevOutput=DiscIntNeverNeededParam  ICPrevScaledInput=DiscIntNeverNeededParam
  Interval Test : simulink/Logic and Bit Operations/Interval Test  IntervalClosedRight=on  uplimit=PLL_lock_window  IntervalClosedLeft=on  lowlimit=-PLL_lock_window  OutDataTypeStr=boolean
  Interval Test1 : simulink/Logic and Bit Operations/Interval Test  IntervalClosedRight=on  uplimit=2*pi*f*(1+PLL_freq_range)  IntervalClosedLeft=on  lowlimit=2*pi*f*(1-PLL_freq_range)  OutDataTypeStr=boolean
  LTI System : Subsystem  BlockChoice=CSS  mask(LTI Block){sys=c2d(tf(1,[1/(f*2*2*pi),1]),Td_es_min), IC=[]}
      mask prompts: sys "LTI system variable"; IC "Initial states (state-space only)"
      mask help:
      | The LTI System block accepts both continuous and discrete LTI models as defined in the Control System Toolbox. Transfer function, state-space, and zero-pole-gain formats are all supported in this block.
      |
      | Note: Initial states are only meaningful for state-space systems.
      mask init:
      | try
      |    % read data to initialize mask variables
      |    [D,Ts,Tdi,Tdo,Tdio,x0,sysname]=...
      |       ltimask('Initialize',gcb,sys,IC);
      |    % update contents
      |    model = bdroot;
      |    df = get_param(model,'dirty');
      |    ltimask('UpdateDiagram',gcb,D,Ts,Tdio);
      |    try      
      |       % Attempt to modify locked library -> error
      |       % Makes block show ??? when loading CSTBLOCKS
      |       % for the first time
      |       set_param(model,'dirty',df)
      |    end
      | catch ME
      |    sys = [];  IC = [];   sysname = '???';
      |    throw(ME)
      | end
      mask Help:
      | The LTI System block accepts any of the three standard LTI models described in the Control System Toolbox: transfer function, zero/pole/gain, or state space. Internally, LTI models will be converted to their state space equivalent for evaluation.
      | <p>
      | In the editable text box labeled <b>LTI System Variable</b>, enter a valid LTI model.
      | <p>
      | In the editable text box labeled <b>Initial States</b> enter the initial state vector.  Initial states are only valid for state-space systems.
      | <p>
      | See also TF, ZPK, SS, LTIMODELS.
      mask CallbackString: ltimask('MaskLTICallback',gcb);|
      mask Display: disp(sysname)
  Logical Operator : Logic  AllPortsSameDT=off  OutDataTypeStr=boolean
  Memory : Memory
  Memory1 : Memory
  PID Controller : simulink/Continuous/PID Controller  Controller=PID  TimeDomain=Discrete-time  SampleTime=PLL_time_step  IntegratorMethod=Forward Euler  FilterMethod=Forward Euler  Form=Parallel  P=PLL_Kp  I=PLL_Ki  D=0  N=100  InitialConditionSource=internal  InitialConditionForIntegrator=2*pi*f  InitialConditionForFilter=0  ExternalReset=none  ZeroCross=off  LimitOutput=on  UpperSaturationLimit=2*pi*(f*(1+PLL_freq_range))  LowerSaturationLimit=2*pi*(f*(1-PLL_freq_range))  LinearizeAsGain=on  AntiWindupMode=clamping  Kb=1  TrackingMode=off  Kt=1  PParamMin=[]  PParamMax=[]  IParamMin=[]  IParamMax=[]  DParamMin=[]  DParamMax=[]  NParamMin=[]  NParamMax=[]  KbParamMin=[]  KbParamMax=[]  KtParamMin=[]  KtParamMax=[]  POutMin=[]  POutMax=[]  IOutMin=[]  IOutMax=[]  DOutMin=[]  DOutMax=[]  NOutMin=[]  NOutMax=[]  KbOutMin=[]  KbOutMax=[]  KtOutMin=[]  KtOutMax=[]  IntegratorOutMin=[]  IntegratorOutMax=[]  FilterOutMin=[]  FilterOutMax=[]  SumOutMin=[]  SumOutMax=[]  SumI1OutMin=[]  SumI1OutMax=[]  SumI2OutMin=[]  SumI2OutMax=[]  SumI3OutMin=[]  SumI3OutMax=[]  SumDOutMin=[]  SumDOutMax=[]  SaturationOutMin=[]  SaturationOutMax=[]  IntegratorContinuousStateAttributes=''  IntegratorStateMustResolveToSignalObject=off  IntegratorRTWStateStorageClass=Auto  FilterContinuousStateAttributes=''  FilterStateMustResolveToSignalObject=off  FilterRTWStateStorageClass=Auto
  Rate Transition : RateTransition  OutPortSampleTime=PLL_time_step
  Subsystem : Subsystem
  Sum : Sum  Inputs=|+-
  Switch : Switch
  Terminator : Terminator
  Terminator1 : Terminator
  Terminator2 : Terminator
  zero : Constant  Value=0
  theta : Outport
  freq : Outport  Port=2
  locked : Outport  Port=3
  wires:
  mode/1 -> Switch/2
  Memory1/1 -> Switch/3
  Switch/1 -> Discrete VCO/1(In1), Memory1/1
  Sum/1 -> PID Controller/1
  LTI System/1(Out1) -> Interval Test/1
  Discrete VCO/2(Sin) -> Terminator1/1
  PID Controller/1 -> Switch/1, freq/1, Interval Test1/1
  Discrete VCO/1(Cos) -> Terminator/1
  Subsystem/1(qd) -> Demux1/1
  abc/1 -> Rate Transition/1
  Interval Test1/1 -> Logical Operator/2
  Interval Test/1 -> Logical Operator/1
  zero/1 -> Sum/2
  Rate Transition/1 -> Subsystem/1(abc)
  Logical Operator/1 -> Data Type Conversion/1
  Discrete VCO/3(theta) -> Subsystem/2(theta), theta/1
  Demux1/1 -> LTI System/1(In1), Memory/1  "Vd"
  Demux1/2 -> Terminator2/1  "Vq"
  Discrete-Time Integrator/1 -> Compare To Constant3/1
  Data Type Conversion/1 -> Compare To Constant1/1, Discrete-Time Integrator/1
  Compare To Constant1/1 -> Discrete-Time Integrator/2
  Compare To Constant3/1 -> locked/1
  Memory/1 -> Sum/1

== system Batt_lib/HIL_BATT/Batt/Grid Tied Inverter/RMS_Calculator ==
  Signal : Inport
  Discrete  Mean value6 : powerlib_extras/Discrete Measurements/Discrete  Mean value  Freq=60/4  Vinit=0  Ts=Ts
  Memory : Memory
  Product3 : Product  RndMeth=Zero
  Signed Sqrt : Sqrt  SaturateOnIntegerOverflow=on
  RMS_Signal : Outport
  wires:
  Signal/1 -> Product3/1, Product3/2
  Product3/1 -> Memory/1
  Discrete  Mean value6/1 -> Signed Sqrt/1
  Signed Sqrt/1 -> RMS_Signal/1
  Memory/1 -> Discrete  Mean value6/1

== system Batt_lib/HIL_BATT/Batt/Grid Tied Inverter/Subsystem ==
  qd : Inport  OutDataTypeStr=double  PortDimensions=2
  theta : Inport  Port=2  OutDataTypeStr=double  PortDimensions=1
  Mux : Mux  Inputs=3
  Mux1 : Mux  Inputs=2
  qd>a : Fcn  Expr=u[1]*cos(u[3])-u[2]*sin(u[3])
  qd>b : Fcn  Expr=u[1]*cos(u[3]-2*pi/3)-u[2]*sin(u[3]-2*pi/3)
  qd>c : Fcn  Expr=u[1]*cos(u[3]+2*pi/3)-u[2]*sin(u[3]+2*pi/3)
  abc : Outport  OutDataTypeStr=double  PortDimensions=3
  wires:
  Mux/1 -> abc/1
  qd>b/1 -> Mux/2
  qd/1 -> Mux1/1
  qd>c/1 -> Mux/3
  theta/1 -> Mux1/2
  Mux1/1 -> qd>c/1, qd>b/1, qd>a/1
  qd>a/1 -> Mux/1

== system Batt_lib/HIL_BATT/Batt/Grid Tied Inverter/Subsystem1 ==
  abc : Inport  OutDataTypeStr=double  PortDimensions=3
  theta : Inport  Port=2  OutDataTypeStr=double  PortDimensions=1
  Mux : Mux  Inputs=2
  Mux1 : Mux  Inputs=2
  abc>d : Fcn  Expr=2/3*(u[1]*cos(u[4])+u[2]*cos(u[4]-2*pi/3)+u[3]*cos(u[4]+2*pi/3))
  abc>q : Fcn  Expr=2/3*(-u[1]*sin(u[4])-u[2]*sin(u[4]-2*pi/3)-u[3]*sin(u[4]+2*pi/3))
  qd : Outport  OutDataTypeStr=double  PortDimensions=2
  wires:
  Mux1/1 -> abc>q/1, abc>d/1
  Mux/1 -> qd/1
  abc>d/1 -> Mux/1
  abc>q/1 -> Mux/2
  theta/1 -> Mux1/2
  abc/1 -> Mux1/1

== system Batt_lib/HIL_BATT/Batt/Grid Tied Inverter/Windowed Limit ==
  Signal : Inport
  Threshold : Inport  Port=2
  Abs : Abs
  Relational Operator2 : RelationalOperator  Operator=>  OutDataTypeStr=boolean
  TestOut : Outport
  wires:
  Abs/1 -> Relational Operator2/1
  Relational Operator2/1 -> TestOut/1
  Threshold/1 -> Relational Operator2/2
  Signal/1 -> Abs/1

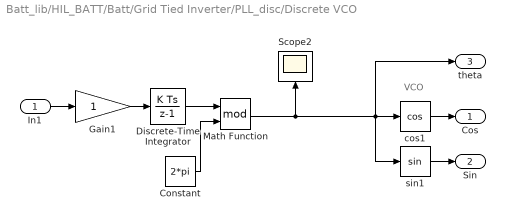
== system Batt_lib/HIL_BATT/Batt/Grid Tied Inverter/PLL_disc/Discrete VCO ==
  note: VCO
  In1 : Inport
  Constant : Constant  Value=2*pi
  Discrete-Time Integrator : DiscreteIntegrator  InitialConditionMode=State only (most efficient)  SampleTime=Td_es_min  ICPrevOutput=DiscIntNeverNeededParam  ICPrevScaledInput=DiscIntNeverNeededParam
  Gain1 : Gain  OutDataTypeStr=double
  Math Function : Math  Operator=mod  SaturateOnIntegerOverflow=on
  Scope2 : Scope
      settings: TimeRange=0.1  YMin=0  YMax=70000
  cos1 : Trigonometry  Operator=cos
  sin1 : Trigonometry
  Cos : Outport
  Sin : Outport  Port=2
  theta : Outport  Port=3
  wires:
  In1/1 -> Gain1/1
  cos1/1 -> Cos/1
  sin1/1 -> Sin/1
  Constant/1 -> Math Function/2
  Gain1/1 -> Discrete-Time Integrator/1
  Discrete-Time Integrator/1 -> Math Function/1
  Math Function/1 -> Scope2/1, theta/1, cos1/1, sin1/1

== system Batt_lib/HIL_BATT/Batt/Grid Tied Inverter/PLL_disc/LTI System ==
  In1 : Inport
  IO Delay : cstextras/Integer Delay (masked)  Td=Tdio  u0=0  Ts=Ts
  Input Delay : cstextras/Integer Delay (masked)  Td=Tdi  u0=0  Ts=Ts
  Internal : DiscreteStateSpace  A=D.a  B=D.b  C=D.c  D=D.d  SampleTime=Ts
  Output Delay : cstextras/Integer Delay (masked)  Td=Tdo  u0=0  Ts=Ts
  Out1 : Outport  InitialOutput=0
  wires:
  IO Delay/1 -> Output Delay/1
  Internal/1 -> IO Delay/1
  Input Delay/1 -> Internal/1
  Output Delay/1 -> Out1/1
  In1/1 -> Input Delay/1

== system Batt_lib/HIL_BATT/Batt/Grid Tied Inverter/PLL_disc/Subsystem ==
  abc : Inport  OutDataTypeStr=double  PortDimensions=3
  theta : Inport  Port=2  OutDataTypeStr=double  PortDimensions=1
  Mux : Mux  Inputs=2
  Mux1 : Mux  Inputs=2
  abc>d : Fcn  Expr=2/3*(u[1]*cos(u[4])+u[2]*cos(u[4]-2*pi/3)+u[3]*cos(u[4]+2*pi/3))
  abc>q : Fcn  Expr=2/3*(-u[1]*sin(u[4])-u[2]*sin(u[4]-2*pi/3)-u[3]*sin(u[4]+2*pi/3))
  qd : Outport  OutDataTypeStr=double  PortDimensions=2
  wires:
  abc/1 -> Mux1/1
  theta/1 -> Mux1/2
  abc>q/1 -> Mux/2
  abc>d/1 -> Mux/1
  Mux/1 -> qd/1
  Mux1/1 -> abc>d/1, abc>q/1

== matlab function HIL_BATT/Batt/Grid Tied Inverter/Idq_con_disc/Vector Saturation ==
  data: u input double; y output double; limit input double; type_sat input double
function y = fcn(u, limit, type_sat)
% When the magnitude is of u is greater than limit prioritize the
% saturation to u(type_sat) dimension.  u is two dimensional input.
%#codegen
y=zeros(2,1); % required initialization
u_sign=sign(u);

if(abs(u(1)) > limit)
    u(1) = u_sign(1).*limit;
end
if(abs(u(2)) > limit)
    u(2) =  u_sign(2).*limit;
end
if(u(1)^2 + u(2)^2 > limit^2)
    if(type_sat == 1) % priority given to u(1)
        y(1) = u(1);
        y(2) = u_sign(2) .* sqrt(limit^2 - u(1)^2); 
    else  % priority given to u(2)
        y(2) = u(2);
        y(1) =  u_sign(1) .* sqrt(limit^2 - u(2)^2); 
    end
else
    y = u;
end
